simulink model "ITireAppMdlSiL"  (R2017b)
settings: Solver=FixedStepAuto  StartTime=0.0  StopTime=10000  FixedStep=0.1  RelTol=1e-3
model workspace (MAT data in the model file):
  AilrflowValidFlag1 = [0.01235 0.03834 0.06233 0.08839 0.11261 0.13833 0.16348 0.18843 0.2134 0.23767 0.26241 0.28847 ... (108920 elements, 54460x2)]
  AilrflowValidFlag2 = [0.01258 0.03858 0.06256 0.08863 0.11285 0.13856 0.16371 0.18866 0.21363 0.2379 0.26264 0.2887 ... (108920 elements, 54460x2)]
  Airflow = [0.01258 0.03858 0.06256 0.08863 0.11285 0.13856 0.16371 0.18866 0.21363 0.2379 0.26264 0.2887 ... (108920 elements, 54460x2)]
  Frequency = [0.01235 0.03834 0.06233 0.08839 0.11261 0.13833 0.16348 0.18843 0.2134 0.23767 0.26241 0.28847 ... (108920 elements, 54460x2)]
  IntkAirHmdty = [0.07576 0.17591 0.27589 0.37591 0.47621 0.5753 0.67605 0.77531 0.87537 0.97532 1.07528 1.17533 ... (27230 elements, 13615x2)]
  IntkAirTemp = [0.07576 0.17591 0.27589 0.37591 0.47621 0.5753 0.67605 0.77531 0.87537 0.97532 1.07528 1.17533 ... (27230 elements, 13615x2)]
  IntkHmdtyTemp = [0.07576 0.17591 0.27589 0.37591 0.47621 0.5753 0.67605 0.77531 0.87537 0.97532 1.07528 1.17533 ... (27230 elements, 13615x2)]
  PriPresFilterValue = [0.01235 0.03834 0.06233 0.08839 0.11261 0.13833 0.16348 0.18843 0.2134 0.23767 0.26241 0.28847 ... (108920 elements, 54460x2)]
  PriPresRawValue = [0.01235 0.03834 0.06233 0.08839 0.11261 0.13833 0.16348 0.18843 0.2134 0.23767 0.26241 0.28847 ... (108920 elements, 54460x2)]
  SecPresFilterValue = [0.01258 0.03858 0.06256 0.08863 0.11285 0.13856 0.16371 0.18866 0.21363 0.2379 0.26264 0.2887 ... (108920 elements, 54460x2)]
  SecPresRawValue = [0.01258 0.03858 0.06256 0.08863 0.11285 0.13856 0.16371 0.18866 0.21363 0.2379 0.26264 0.2887 ... (108920 elements, 54460x2)]
  deltaPriPresFilterV = [0.01235 0.03834 0.06233 0.08839 0.11261 0.13833 0.16348 0.18843 0.2134 0.23767 0.26241 0.28847 ... (108920 elements, 54460x2)]
  deltaPriPresRawValu = [0.01235 0.03834 0.06233 0.08839 0.11261 0.13833 0.16348 0.18843 0.2134 0.23767 0.26241 0.28847 ... (108920 elements, 54460x2)]
  deltaSecPresFilterV = [0.01258 0.03858 0.06256 0.08863 0.11285 0.13856 0.16371 0.18866 0.21363 0.2379 0.26264 0.2887 ... (108920 elements, 54460x2)]
  deltaSecPresRawValu = [0.01258 0.03858 0.06256 0.08863 0.11285 0.13856 0.16371 0.18866 0.21363 0.2379 0.26264 0.2887 ... (108920 elements, 54460x2)]
undefined symbols (not defined in the file or in its folder): sigbuilder_block
(part 2 of 2)

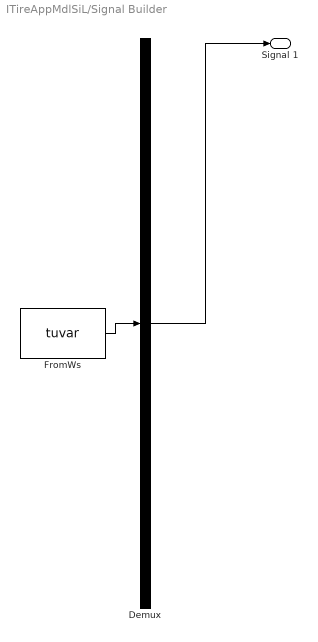
== system ITireAppMdlSiL/Signal Builder ==
  Demux : Demux  Tag=STV Demux  Outputs=1
  FromWs : FromWorkspace  Tag=STV FromWs  VariableName=tuvar  SampleTime=0
      SigBuilderData=|
      | common.afterFinalStr = 'Extrapolate'
      | common.sampleTime = 0
      | dataSet.timeRange = [0 10000]
      | dataSet.name = 'Group 1'
      | sbobj.Groups.Name = 'Group 1'
      | sbobj.Groups.Signals.Name = 'Signal 1'
      | sbobj.Groups.Signals.XData = [0 100 9990 9990 9999 10000]
      | sbobj.Groups.Signals.YData = [280 238 238 22 44 0]
      | sbobj.Groups.TimeRange = [0 10000]
  Signal 1 : Outport  Tag=STV Outport
  wires:
  Demux/1 -> Signal 1/1
  FromWs/1 -> Demux/1

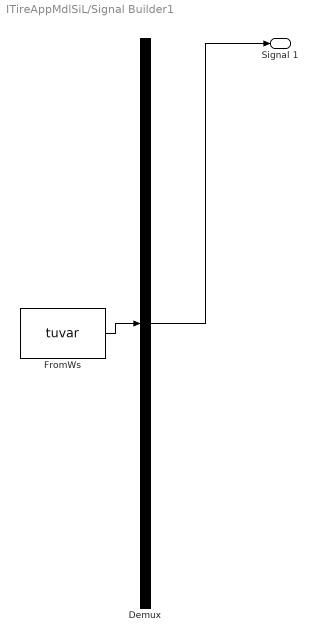
== system ITireAppMdlSiL/Signal Builder1 ==
  Demux : Demux  Tag=STV Demux  Outputs=1
  FromWs : FromWorkspace  Tag=STV FromWs  VariableName=tuvar  SampleTime=0
      SigBuilderData=|
      | common.afterFinalStr = 'Extrapolate'
      | common.sampleTime = 0
      | dataSet.timeRange = [0 10000]
      | dataSet.name = 'Group 1'
      | sbobj.Groups.Name = 'Group 1'
      | sbobj.Groups.Signals.Name = 'Signal 1'
      | sbobj.Groups.Signals.XData = [0 60 9990 9990 9999 10000]
      | sbobj.Groups.Signals.YData = [250 200 118 22 44 0]
      | sbobj.Groups.TimeRange = [0 10000]
  Signal 1 : Outport  Tag=STV Outport
  wires:
  FromWs/1 -> Demux/1
  Demux/1 -> Signal 1/1

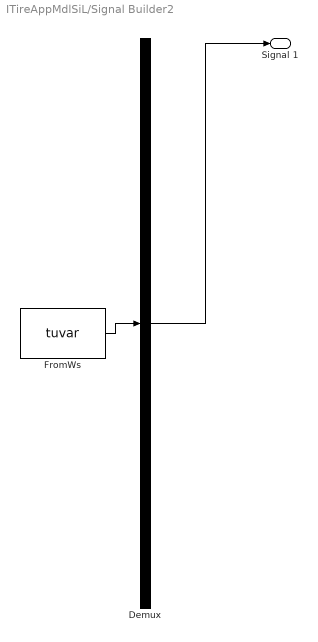
== system ITireAppMdlSiL/Signal Builder2 ==
  Demux : Demux  Tag=STV Demux  Outputs=1
  FromWs : FromWorkspace  Tag=STV FromWs  VariableName=tuvar  SampleTime=0
      SigBuilderData=|
      | common.afterFinalStr = 'Extrapolate'
      | common.sampleTime = 0
      | dataSet.timeRange = [0 10000]
      | dataSet.name = 'Group 1'
      | sbobj.Groups.Name = 'Group 1'
      | sbobj.Groups.Signals.Name = 'Signal 1'
      | sbobj.Groups.Signals.XData = [0 60 9990 9990 9999 10000]
      | sbobj.Groups.Signals.YData = [250 248 80 22 44 0]
      | sbobj.Groups.TimeRange = [0 10000]
  Signal 1 : Outport  Tag=STV Outport
  wires:
  Demux/1 -> Signal 1/1
  FromWs/1 -> Demux/1

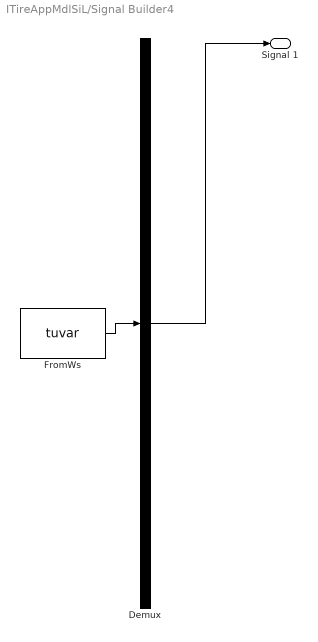
== system ITireAppMdlSiL/Signal Builder4 ==
  Demux : Demux  Tag=STV Demux  Outputs=1
  FromWs : FromWorkspace  Tag=STV FromWs  VariableName=tuvar  SampleTime=0
      SigBuilderData=|
      | common.afterFinalStr = 'Extrapolate'
      | common.sampleTime = 0
      | dataSet.timeRange = [0 10000]
      | dataSet.name = 'Group 1'
      | sbobj.Groups.Name = 'Group 1'
      | sbobj.Groups.Signals.Name = 'Signal 1'
      | sbobj.Groups.Signals.XData = [0 9999 10000]
      | sbobj.Groups.Signals.YData = [380 350 350]
      | sbobj.Groups.TimeRange = [0 10000]
  Signal 1 : Outport  Tag=STV Outport
  wires:
  FromWs/1 -> Demux/1
  Demux/1 -> Signal 1/1
